simulink model "sys_dae_dos"  (R2021a)
settings: Solver=ode23t  StartTime=0.0  StopTime=20  RelTol=1e-3
settings Model: Creator=Suman  LastModifiedBy=Suman

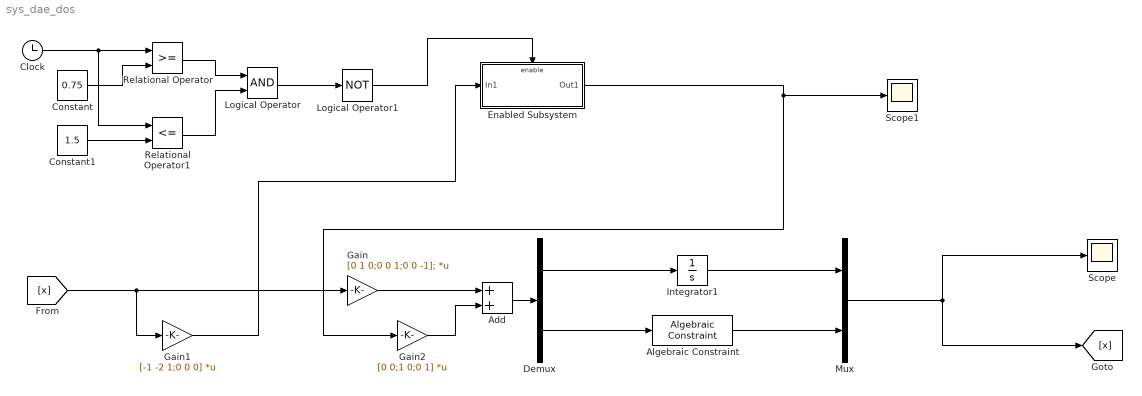
== system sys_dae_dos ==
  Add : Sum
  Algebraic Constraint : AlgebraicConstraint
  Clock : Clock
  Constant : Constant  Value=0.75
  Constant1 : Constant  Value=1.5
  Demux : Demux  Outputs=2
  Enabled Subsystem : Subsystem  TreatAsAtomicUnit=on
  Gain : Gain  Gain=[0 1 0;0 0 1;0 0 -1];  Multiplication=Matrix(K*u) (u vector)
  Gain1 : Gain  Gain=[-1 -2 1;0 0 0]  Multiplication=Matrix(K*u) (u vector)
  Gain2 : Gain  Gain=[0 0;1 0;0 1]  Multiplication=Matrix(K*u) (u vector)
  Integrator1 : Integrator  InitialCondition=[2;3]
  Logical Operator : Logic  AllPortsSameDT=off  OutDataTypeStr=boolean
  Logical Operator1 : Logic  Operator=NOT  AllPortsSameDT=off  OutDataTypeStr=boolean
  Mux : Mux  Inputs=2
  Relational Operator : RelationalOperator  OutDataTypeStr=boolean  RndMeth=Simplest
  Relational Operator1 : RelationalOperator  Operator=<=  OutDataTypeStr=boolean  RndMeth=Simplest
  Scope : Scope
  Scope1 : Scope
  wires:
  Enabled Subsystem/1(Out1) -> Gain2/1, Scope1/1
  Constant/1 -> Relational Operator/2
  Relational Operator1/1 -> Logical Operator/2
  Relational Operator/1 -> Logical Operator/1
  Constant1/1 -> Relational Operator1/2
  Clock/1 -> Relational Operator1/1, Relational Operator/1
  [x] -> Gain1/1, Gain/1
  Gain/1 -> Add/1
  Demux/1 -> Integrator1/1
  Mux/1 -> [x], Scope/1
  Algebraic Constraint/1 -> Mux/2
  Gain2/1 -> Add/2
  Demux/2 -> Algebraic Constraint/1
  Add/1 -> Demux/1
  Integrator1/1 -> Mux/1
  Logical Operator/1 -> Logical Operator1/1
  Logical Operator1/1 -> Enabled Subsystem/Enable
  Gain1/1 -> Enabled Subsystem/1(In1)

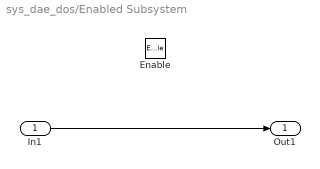
== system sys_dae_dos/Enabled Subsystem ==
  In1 : Inport
  Enable : EnablePort
  Out1 : Outport
  wires:
  In1/1 -> Out1/1
